simulink model "question2"  (R2016b)
settings: Solver=FixedStepAuto  StartTime=0.0  StopTime=pi*8  FixedStep=0.01  RelTol=1e-3
libraries: simulink x1, fuzblock x1
settings Model: Creator=Dreamer  LastModifiedBy=Dreamer

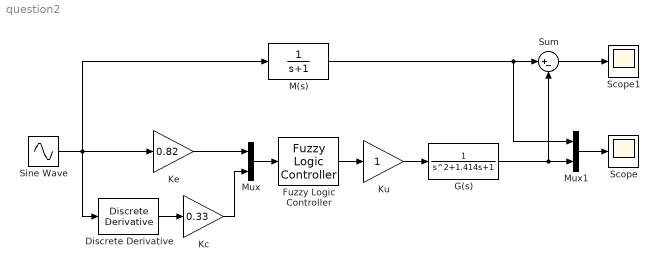
== system question2 ==
  Discrete Derivative : simulink/Discrete/Discrete Derivative  gainval=1.0  ICPrevScaledInput=0.0  OutMin=[]  OutMax=[]  OutDataType=fixdt(1, 16)  OutScaling=2^-10  DoSatur=off
  Fuzzy Logic Controller : fuzblock/Fuzzy Logic  Controller  fis='question1.fis'
  G(s) : TransferFcn  Denominator=[1 1.414 1]
  Kc : Gain  Gain=0.33
  Ke : Gain  Gain=0.82
  Ku : Gain
  M(s) : TransferFcn  Denominator=[1 1]
  Mux : Mux  Inputs=2
  Mux1 : Mux  Inputs=2
  Scope : Scope
  Scope1 : Scope
  Sine Wave : Sin  Frequency=0.5  SampleTime=0
  Sum : Sum  Inputs=|+-
  wires:
  Ke/1 -> Mux/1
  Kc/1 -> Mux/2
  Mux/1 -> Fuzzy Logic Controller/1
  Fuzzy Logic Controller/1 -> Ku/1
  Ku/1 -> G(s)/1
  Sine Wave/1 -> M(s)/1, Discrete Derivative/1, Ke/1
  Mux1/1 -> Scope/1
  G(s)/1 -> Mux1/2, Sum/2
  M(s)/1 -> Sum/1, Mux1/1
  Discrete Derivative/1 -> Kc/1
  Sum/1 -> Scope1/1
